simulink model "Phone_B"  (R2023a)
settings: Solver=FixedStepDiscrete  StartTime=0.0  StopTime=inf  RelTol=1e-3
libraries: androidcommunicationlib x6, androiduilib x6, androidaudiovideolib x2
settings Model: Creator=patel  LastModifiedBy=patel
settings OptimizationCC: EnhancedBackFolding=on  PassReuseOutputArgsAs=Individual arguments  ZeroExternalMemoryAtStartup=off  ZeroInternalMemoryAtStartup=off  MaxStackSize=64  OptimizeBlockOrder=speed  DifferentSizesBufferReuse=on  OptimizationCustomize=off  EfficientTunableParamExpr=on
settings DebuggingCC: ParameterTunabilityLossMsg=error
settings HardwareCC: ProdBitPerPointer=32  ProdBitPerSizeT=32  ProdBitPerPtrDiffT=32  ProdLargestAtomicInteger=Long  ProdLargestAtomicFloat=Double  ProdWordSize=32  ProdHWDeviceType=ARM Compatible->ARM Cortex  UseEmbeddedCoderFeatures=off  UseSimulinkCoderFeatures=off
settings SFSimCC: MATLABDynamicMemAlloc=off
settings RTWCC: Description=Embedded Coder  SystemTargetFile=ert.tlc  HardwareBoard=Android Device  TLCOptions="-aInlineSetEventsForThisBaseRateFcn=TLC_FALSE -aSuppressMultiTaskScheduler=TLC_FALSE  -aRateBasedStepFcn=0"  TemplateMakefile=ert_default_tmf  RTWVerbose=off  Toolchain=Android SDK/NDK Tools
settings CodeAppCC: ForceParamTrailComments=on  IgnoreCustomStorageClasses=off  OperatorAnnotations=on  SimulinkDataObjDesc=on  SFDataObjDesc=on  InsertBlockDesc=on
settings ERTTargetCC: SupportNonInlinedSFcns=on

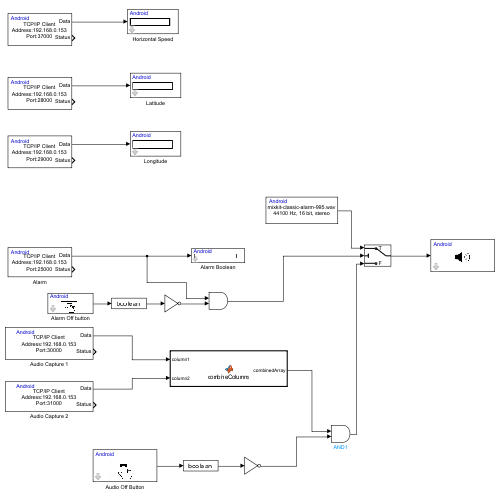
[thumbnail: Simulink's stored preview of the top-level diagram]
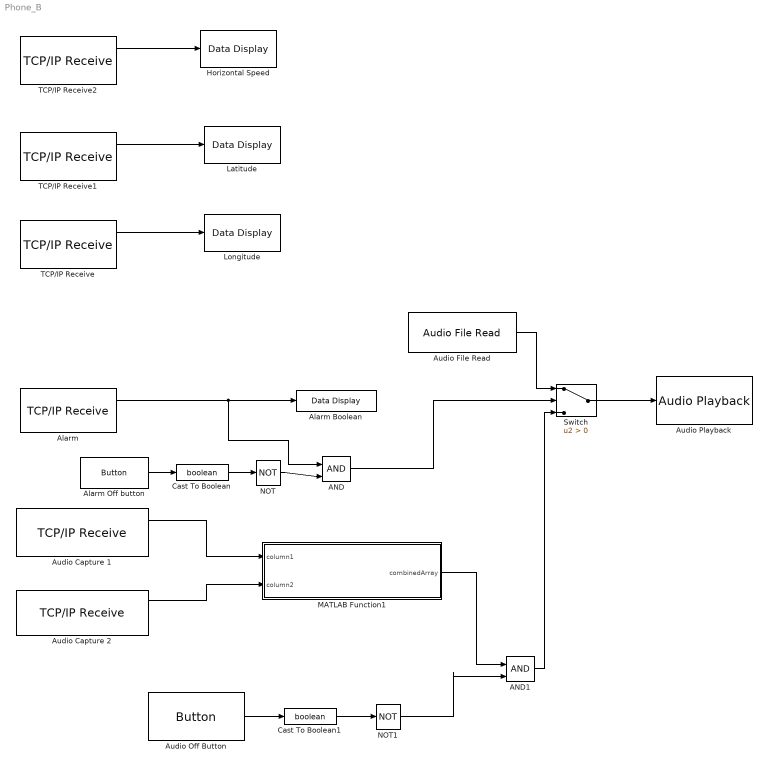
== system Phone_B ==
  AND : Logic  IconShape=distinctive  AllPortsSameDT=off  OutDataTypeStr=boolean
  AND1 : Logic  IconShape=distinctive  AllPortsSameDT=off  OutDataTypeStr=boolean
  Alarm : androidcommunicationlib/TCP//IP Receive  TCPReceiveId=Phone_B/Alarm  Mode_=Client  LocalServerPort_=25000  RemoteAddr_=192.168.0.153  RemoteServerPort_=25000  DataType_=uint8  DataSize_=1  SampleTime_=0.1  ClientPortBindingSelection_=off  ClientPortToBind_=35000  BlockingMode_=off  BlockTimeout_=0.1
  Alarm Boolean : androiduilib/Data Display  DataDisplayId=Phone_B/Alarm_Boolean  Format=Float  Precision=6  SimulateUsing=Code generation  blockPlatform=Android
  Alarm Off button : androiduilib/Button  ButtonState=Not pressed  ButtonId=Phone_B/Alarm_Off_button  State=off  SampleTime=0.1  BlockPlatform=Android
  Audio Capture 1 : androidcommunicationlib/TCP//IP Receive  TCPReceiveId=Phone_B/Audio_Capture_1  Mode_=Client  LocalServerPort_=25000  RemoteAddr_=192.168.0.153  RemoteServerPort_=30000  DataType_=int16  DataSize_=4410  SampleTime_=0.1  ClientPortBindingSelection_=off  ClientPortToBind_=35000  BlockingMode_=off  BlockTimeout_=0.1
  Audio Capture 2 : androidcommunicationlib/TCP//IP Receive  TCPReceiveId=Phone_B/Audio_Capture_2  Mode_=Client  LocalServerPort_=25000  RemoteAddr_=192.168.0.153  RemoteServerPort_=31000  DataType_=int16  DataSize_=4410  SampleTime_=0.1  ClientPortBindingSelection_=off  ClientPortToBind_=35000  BlockingMode_=off  BlockTimeout_=0.1
  Audio File Read : androidaudiovideolib/Audio File Read  FileName=C:\Users\patel\Downloads\mixkit-classic-alarm-995.wav  FrameSize=4410
  Audio Off Button : androiduilib/Button  ButtonState=Not pressed  ButtonId=Phone_B/Audio_Off_Button  State=off  SampleTime=0.1  BlockPlatform=Android
  Audio Playback : androidaudiovideolib/Audio Playback  SampleFreq=44100  AudioSamplingFreq=44100  SampleTime=0.1  DeviceStr=0  QueueDuration=0  BlockPlatform=Android
  Cast To Boolean : DataTypeConversion  OutDataTypeStr=boolean  SaturateOnIntegerOverflow=off  RndMeth=Floor
  Cast To Boolean1 : DataTypeConversion  OutDataTypeStr=boolean  SaturateOnIntegerOverflow=off  RndMeth=Floor
  Horizontal Speed : androiduilib/Data Display  DataDisplayId=Phone_B/Horizontal_Speed  Format=Float  Precision=6  SimulateUsing=Code generation  blockPlatform=Android
  Latitude : androiduilib/Data Display  DataDisplayId=Phone_B/Latitude  Format=Float  Precision=6  SimulateUsing=Code generation  blockPlatform=Android
  Longitude : androiduilib/Data Display  DataDisplayId=Phone_B/Longitude  Format=Float  Precision=6  SimulateUsing=Code generation  blockPlatform=Android
  MATLAB Function1 : MATLAB Function  TreatAsAtomicUnit=on
  NOT : Logic  Operator=NOT  IconShape=distinctive  AllPortsSameDT=off  OutDataTypeStr=boolean
  NOT1 : Logic  Operator=NOT  IconShape=distinctive  AllPortsSameDT=off  OutDataTypeStr=boolean
  Switch : Switch  Criteria=u2 > Threshold  OutDataTypeStr=int16  SaturateOnIntegerOverflow=off  InputSameDT=off
  TCP/IP Receive : androidcommunicationlib/TCP//IP Receive  TCPReceiveId=Phone_B/TCP//IP_Receive  Mode_=Client  LocalServerPort_=25000  RemoteAddr_=192.168.0.153  RemoteServerPort_=29000  DataType_=double  DataSize_=1  SampleTime_=2  ClientPortBindingSelection_=off  ClientPortToBind_=35000  BlockingMode_=off  BlockTimeout_=0.1
  TCP/IP Receive1 : androidcommunicationlib/TCP//IP Receive  TCPReceiveId=Phone_B/TCP//IP_Receive1  Mode_=Client  LocalServerPort_=25000  RemoteAddr_=192.168.0.153  RemoteServerPort_=28000  DataType_=double  DataSize_=1  SampleTime_=2  ClientPortBindingSelection_=off  ClientPortToBind_=35000  BlockingMode_=off  BlockTimeout_=0.1
  TCP/IP Receive2 : androidcommunicationlib/TCP//IP Receive  TCPReceiveId=Phone_B/TCP//IP_Receive2  Mode_=Client  LocalServerPort_=25000  RemoteAddr_=192.168.0.153  RemoteServerPort_=37000  DataType_=uint8  DataSize_=1  SampleTime_=0.1  ClientPortBindingSelection_=off  ClientPortToBind_=35000  BlockingMode_=off  BlockTimeout_=0.1
  wires:
  Alarm/1 -> AND/1, Alarm Boolean/1
  Audio Capture 1/1 -> MATLAB Function1/1(column1)
  Audio Capture 2/1 -> MATLAB Function1/2(column2)
  MATLAB Function1/1(combinedArray) -> AND1/1
  TCP/IP Receive/1 -> Longitude/1
  TCP/IP Receive1/1 -> Latitude/1
  Audio File Read/1 -> Switch/1
  Switch/1 -> Audio Playback/1
  Alarm Off button/1 -> Cast To Boolean/1
  Cast To Boolean/1 -> NOT/1
  NOT/1 -> AND/2
  AND/1 -> Switch/2
  TCP/IP Receive2/1 -> Horizontal Speed/1
  Audio Off Button/1 -> Cast To Boolean1/1
  Cast To Boolean1/1 -> NOT1/1
  NOT1/1 -> AND1/2
  AND1/1 -> Switch/3

== matlab function Phone_B/MATLAB Function1 ==
  data: column1 input; combinedArray output; column2 input
function combinedArray = combineColumns(column1, column2)

    % Combine the two columns into an Nx2 array
    combinedArray = [column1(:), column2(:)];
end
